simulink model "stellaris_lp_loopback"  (R2017a)
settings: Solver=ode3  StartTime=0.0  StopTime=inf  FixedStep=0.005  RelTol=1e-3
libraries: stellaris_lp_lib x3, xpcutilitieslib x2
settings Model: ExtModeTrigDuration=2  Creator=peselnikmg  LastModifiedBy=Nilim
settings DataIOCC: LimitDataPoints=on  SaveFormat=Array  SignalLoggingSaveFormat=ModelDataLogs
settings OptimizationCC: PassReuseOutputArgsAs=Individual arguments  ExpressionDepthLimit=2147483647  MaxStackSize=64
settings DebuggingCC: ParameterTunabilityLossMsg=error  StateNameClashWarn=warning  SFUnexpectedBacktrackingDiag=warning  SFNoUnconditionalDefaultTransitionDiag=warning  SFExecutionAtInitializationDiag=none
settings HardwareCC: ProdBitPerPointer=32  ProdBitPerSizeT=32  ProdBitPerPtrDiffT=32  ProdLargestAtomicInteger=Long  ProdLargestAtomicFloat=Double  ProdWordSize=32  ProdHWDeviceType=ARM Compatible->ARM Cortex
settings ModelReferenceCC: PropagateSignalLabelsOutOfModel=off
settings SFSimCC: MATLABDynamicMemAlloc=off
settings RTWCC: SystemTargetFile=ert.tlc  HardwareBoard=Tiva TM4C123G Launchpad  TLCOptions=-aInlineSetEventsForThisBaseRateFcn=TLC_FALSE -aSuppressMultiTaskScheduler=TLC_FALSE -aRateBasedStepFcn=1  TemplateMakefile=ert_default_tmf  Description=Embedded Coder  GenerateReport=on  RTWVerbose=off  Toolchain=Texas Instruments Code Composer Studio (Tiva)  IncludeHyperlinkInReport=on  LaunchReport=on  GenerateTraceInfo=on  GenerateTraceReport=on  GenerateTraceReportSl=on  GenerateTraceReportSf=on  GenerateTraceReportEml=on
settings CodeAppCC: ForceParamTrailComments=on  IgnoreCustomStorageClasses=off  OperatorAnnotations=on  SimulinkDataObjDesc=on  SFDataObjDesc=on  MATLABFcnDesc=on  CustomSymbolStrType=$N$R$M  InsertBlockDesc=on  MATLABSourceComments=on  InternalIdentifier=Classic
settings ERTTargetCC: SupportContinuousTime=on
settings ConfigComp: CovMetricSettings=dw  CovHtmlReporting=on  CovSaveCumulativeToWorkspaceVar=on  CovSaveSingleToWorkspaceVar=on  CovExternalEMLEnable=off

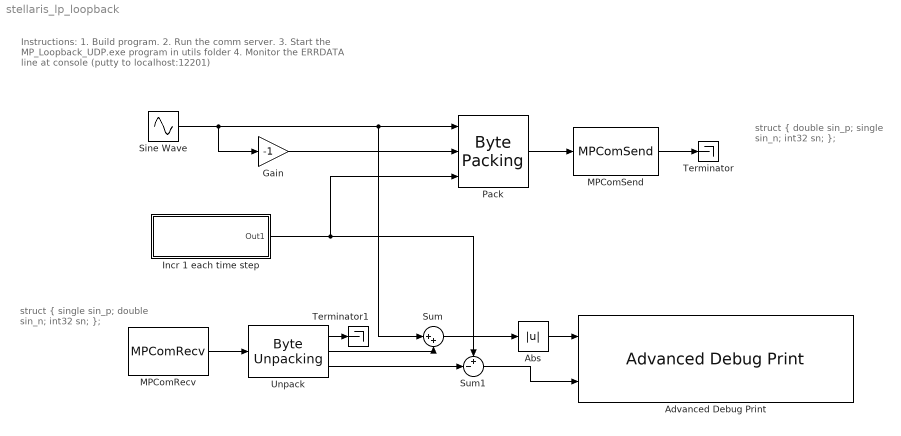
== system stellaris_lp_loopback ==
  note: Instructions:
      | 1. Build program.
      | 2. Run the comm server.
      | 3. Start the MP_Loopback_UDP.exe program in utils folder
      | 4. Monitor the ERRDATA line at console (putty to localhost:12201)
  note: struct  {
      | 		double sin_p;
      | 		single sin_n;
      | 		int32 sn;
      | };
  note: struct  {
      | 		single sin_p;
      | 		double sin_n;
      | 		int32 sn;
      | };
  Abs : Abs
  Advanced Debug Print : stellaris_lp_lib/Debug/Advanced Debug Print  types={'double','int32'}  fmt='ERRDATA %f %d\r\n'  sample_time=0.05
      settings: SourceProductName=Run on Stellaris LaunchPad
  Gain : Gain  Gain=-1  OutDataTypeStr=single
  Incr 1 each time step : Subsystem
  MPComRecv : stellaris_lp_lib/Communication/MPComRecv  vport=3  pack_size=16  sample_time=0.005
      settings: SourceProductName=Run on Stellaris LaunchPad
  MPComSend : stellaris_lp_lib/Communication/MPComSend  vport=2  pack_size=16  sample_time=0.005
      settings: SourceProductName=Run on Stellaris LaunchPad
  Pack : xpcutilitieslib/Byte Packing   MaskPackedDataType=uint8  MaskUnpackedDataTypes={'double','single','int32'}  MaskAlignment=1
  Sine Wave : Sin  SampleTime=0
  Sum : Sum  Inputs=|++
  Sum1 : Sum  Inputs=+-|
  Terminator : Terminator
  Terminator1 : Terminator
  Unpack : xpcutilitieslib/Byte Unpacking   MaskUnpackedDataTypes={'single','double', 'int32'}  MaskUnpackedDataSizes={[1],[1],[1]}  MaskAlignment=1
      settings: SourceProductName=Simulink Real-Time  SourceProductBaseCode=XP
  wires:
  MPComRecv/1 -> Unpack/1
  Pack/1 -> MPComSend/1
  Gain/1 -> Pack/2
  Sine Wave/1 -> Gain/1, Sum/1, Pack/1
  MPComSend/1 -> Terminator/1
  Unpack/2 -> Sum/2
  Unpack/3 -> Sum1/2
  Sum1/1 -> Advanced Debug Print/2
  Incr 1 each time step/1(Out1) -> Pack/3, Sum1/1
  Sum/1 -> Abs/1
  Unpack/1 -> Terminator1/1
  Abs/1 -> Advanced Debug Print/1

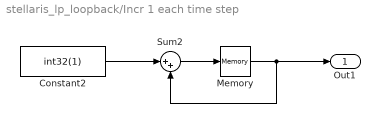
== system stellaris_lp_loopback/Incr 1 each time step ==
  Constant2 : Constant  Value=int32(1)  SampleTime=-1
  Memory : Memory
  Sum2 : Sum  Inputs=|++
  Out1 : Outport  PortDimensions=1
  wires:
  Constant2/1 -> Sum2/1
  Sum2/1 -> Memory/1
  Memory/1 -> Out1/1, Sum2/2
